simulink model "sbc_uja1169_rw_reg_s32k11x"  (Simulink 9.0)
settings: Solver=FixedStepDiscrete  StartTime=0.0  StopTime=10.0  FixedStep=0.1  RelTol=1e-3  EnableMultiTasking=on
InitFcn:
  | mbd_s32k_consistency_checks(bdroot(gcs));
undefined symbols (not defined in the file): bit, F, LQFP, thumb, UJA1169TK
libraries: mbd_s32k1xx_ec_toolbox x6, mbd_sbc_ec_toolbox x5, simulink x3
Description:
  | This model shows how to use SBC_Read_Register and SBC_Write_Register blocks.
  | The SBC is configured with reset threshold set to 90 % of V1 nominal output voltage, and after several seconds the reset threshold is set to 60% of V1 .
  | 
  | 
  | Validation:
  |  - RED Led should be on about 5 sec (reset threshold set to 90 %)
  | -  BLUE Led should be on after more than 5 sec (reset threshold set to 60 %)
  | 
  | Notes:
  | The test requires correct factory settings: FNMC bit disabled, SBC_UJA_SBC_SDMC_DIS disabled and slpc must be allowed.
  | For running other applications is recommended to move the SBC in FNMC after running this example,
  | otherwise CAN transceiver can be disabled because SBC goes in LIMP mode due to lack of watchdog feed.
  | 
  | To move SBC in FNMC state:
  |    - pin RSTN (TP24) is held LOW
  |    -CANH is pulled up to Vbat
  |    -CANL is pulled down to GND
  | 
  | 
  | HW prerequisite:
  | - S32K116/S32K118
  | - One Power Adapter 12V
settings Model: Creator=NXP MBDT Team  LastModifiedBy=nxf35172
settings DataIOCC: ExternalInput=off  InitialState=off  SaveFormat=Dataset  SaveOutput=off  SignalLogging=off  SaveTime=off
settings OptimizationCC: DefaultParameterBehavior=Inlined  LifeSpan=1
settings DebuggingCC: UnderspecifiedInitializationDetection=Simplified  MergeDetectMultiDrivingBlocksExec=error  InheritedTsInSrcMsg=none  SingleTaskRateTransMsg=error  UnconnectedInputMsg=error  UnconnectedOutputMsg=error  UnconnectedLineMsg=error  UnknownTsInhSupMsg=error
settings HardwareCC: ProdLargestAtomicInteger=Long  ProdLargestAtomicFloat=Double  ProdIntDivRoundTo=Zero  ProdEndianess=LittleEndian  ProdHWDeviceType=ARM Compatible->ARM Cortex
settings ModelReferenceCC: PropagateSignalLabelsOutOfModel=on
settings SFSimCC: MATLABDynamicMemAlloc=off
settings RTWCC: SystemTargetFile=mbd_s32k.tlc  MakeCommand=mbd_s32k_make_rtw COPY_MDLREF_INCLUDES=0  TemplateMakefile=mbd_s32k.tmf  Description=Model Based Design Toolbox S32K14x Code Generation Target  GenerateReport=on  IncludeHyperlinkInReport=on  LaunchReport=on  GenerateTraceInfo=on  GenerateTraceReport=on  GenerateTraceReportSl=on  GenerateTraceReportSf=on  GenerateTraceReportEml=on
settings CodeAppCC: ForceParamTrailComments=on  IgnoreCustomStorageClasses=off  OperatorAnnotations=on  SimulinkDataObjDesc=on  SFDataObjDesc=on  MATLABFcnDesc=on  InsertBlockDesc=on  MATLABSourceComments=on
settings STFCustomTargetCC: CombineOutputUpdateFcns=on  ERTCustomFileBanners=on  SupportContinuousTime=off  SupportNonInlinedSFcns=off  RemoveResetFunc=on  MATLABClassNameForMDSCustomization=Simulink.SoftwareTarget.ERTCustomization  GRTInterface=off  SystemTargetFile=mbd_s32k.tlc
settings ERTTargetCC: MultiwordLength=2048  ParMdlRefBuildCompliant=off  CompOptLevelCompliant=off  ConcurrentExecutionCompliant=off  ModelStepFunctionPrototypeControlCompliant=off  CPPClassGenCompliant=off  UseToolchainInfoCompliant=off  InlinedParameterPlacement=NonHierarchical  ERTCustomFileTemplate=example_file_process.tlc

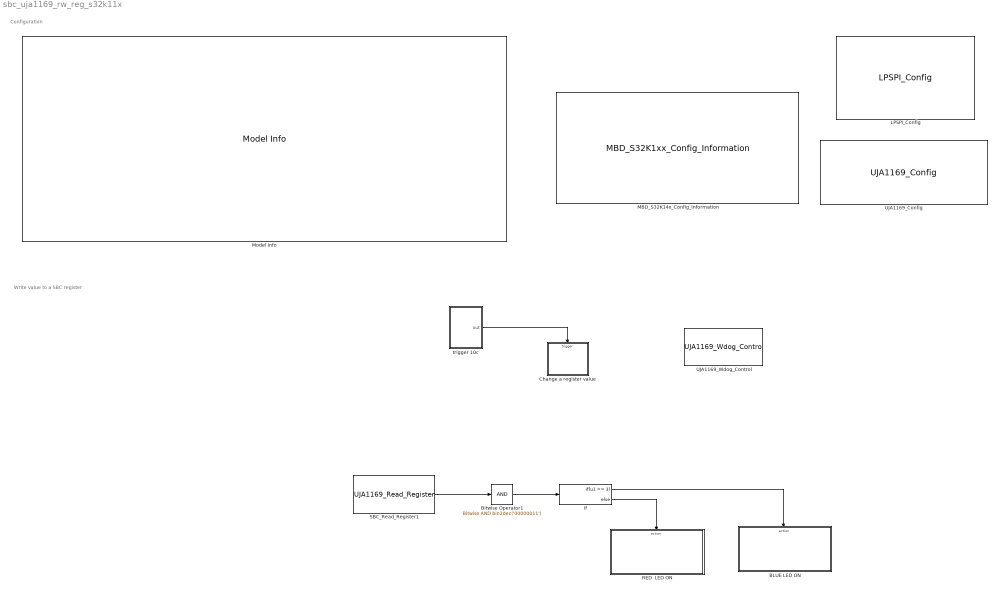
== system sbc_uja1169_rw_reg_s32k11x ==
  note: Configuration
  note: Write value to a SBC register
  BLUE LED ON : Subsystem  TreatAsAtomicUnit=on
  Bitwise Operator1 : simulink/Logic and Bit Operations/Bitwise Operator  logicop=AND  UseBitMask=on  BitMask=bin2dec('00000011')  BitMaskRealWorld=Stored Integer
  Change a register value : Subsystem
  If : If  IfExpression=u1 == 3
  "LPSPI_Config " : mbd_s32k1xx_ec_toolbox/Communication Blocks/SPI Blocks/LPSPI_Config   Priority=1  InstanceNumber=0  Role=Master  BaudRate=50000  ShowAdvanced=on  sin=PTB3: [LPSPI0_SIN | LPSPI Serial Data Input]  sout=PTB4: [LPSPI0_SOUT | LPSPI Serial Data Output]  sck=PTB2: [LPSPI0_SCK | LPSPI Serial Clock I/O]  pcs0=None  pcs1=PTB5: [LPSPI0_PCS1 | Peripheral Chip Select 1]  pcs2=None  pcs3=not available  CPHA=1  CPOL=0  BitOrder=MSB first  TransferSize=16  WhichPCS=1  PCSPol=ActiveLow  ContinuousTransfer=off
  MBD_S32K14x_Config_Information : mbd_s32k1xx_ec_toolbox/MBD_S32K1xx_Config_Information  Priority=0  mbdt_ver=0  disp_str=|  config_params=[]  mcu_target_name=S32K118  mcu_target_package=48-LQFP  mcu_target_sram_size=25KB  mcu_system_clock_freq=40  mcu_xtal_freq=External 40  mcu_steptick_timer=LPIT Channel 0  mcu_steptick_prio=3  ds_import_enable=on  target_compiler=GCC  target_memory=FLASH  gcc_target_compile_opts=-mcpu=cortex-m0plus -mthumb -O1 -g -gstrict-dwarf  gcc_target_assemble_opts=-mcpu=cortex-m0plus -mthumb -g  gcc_target_link_opts=-mcpu=cortex-m0plus -mthumb  gcc_target_default_lcf=on  gcc_target_user_lcf=S32K118_25_flash.ld  ghs_target_compile_opts=-mcpu=cortexm0plus -mthumb -fsoft -Ogeneral -Wundef -Wimplicit-int -Wshadow -Wtrigraphs --no_commons --gnu_asm -gnu99 -gdwarf-2 -G  ghs_target_assemble_opts=-mcpu=cortexm0plus -mthumb -fsoft --gnu_asm  ghs_target_link_opts=-mcpu=cortexm0plus -mthumb -fsoft  ghs_target_default_lcf=off  ghs_target_user_lcf=S32K118_25_flash.ld  iar_target_compile_opts=--thumb -Ol -e --debug --dlib_config normal  iar_target_assemble_opts=--thumb  iar_target_link_opts=--no_exceptions --vfe --inline  iar_target_default_lcf=off  iar_target_user_lcf=S32K118_25_flash.icf  pil_download_enable=off  rbl_download_enable=on  rbl_start_delay=5000000  rbl_download_interface=OpenSDA  rbl_restart_request=off  rbl_com_port=Custom  rbl_com_port_custom=COM1  pil_download_rate=57600  pil_opensda_drive=Custom  pil_opensda_drive_custom=D  pil_uart_instance=0  pil_uart_rx=PTA2: [LPUART0_RX | Receive]  pil_uart_tx=PTA3: [LPUART0_TX | Transmit]  FTM_PWM_PcrCheckEnDis=on  FTM_Input_Edge_Inputs_PcrCheckEnDis=off  FTM_Dual_Edge_Inputs_PcrCheckEnDis=off  FTM_Quadrature_Inputs_PcrCheckEnDis=off  FTM_Hall_Sensor_Inputs_PcrCheckEnDis=on  LPTMR_PcrCheckEnDis=off  PIT_PcrCheckEnDis=off  RTC_PcrCheckEnDis=off  FlexCAN_PcrCheckEnDis=off  LIN_PcrCheckEnDis=on  FlexIO_PcrCheckEnDis=off  LPI2C_PcrCheckEnDis=off  LPSPI_PcrCheckEnDis=on  LPUART_PcrCheckEnDis=off  CMP_PcrCheckEnDis=off  GPIO_OutputPcrCheckEnDis=on  GPIO_InputPcrCheckEnDis=on  SBC_PcrCheckEnDis=on  AMMCLIB_PcrCheckEnDis=off  FM_PcrCheckEnDis=off  Profile_PcrCheckEnDis=off  ConfigParams_PcrCheckEnDis=on  ModelRef_PcrCheckEnDis=on  PDB0_PcrCheckEnDis=off  CSEc_PcrCheckEnDis=off  eDMA_PcrCheckEnDis=off  ADC_PcrCheckEnDis=off  WDOG_PcrCheckEnDis=on
      | Target : S32K144-64KB_SRAM
      | Package : 100-pin
      | System clock : 80 MHz
      | XTAL clock : External 8 MHz
      | Compiler : IAR
      | Target Type : FLASH
      | Download Code after build : off
      | Step Tick Interrupt Priority : 15
  Model Info : simulink/Model-Wide Utilities/Model Info  Frame=off  DisplayStringWithTags=|  HorizontalTextAlignment=Left  LeftAlignmentValue=0.02
      | Model Name: %<ModelName>
      | 
      | Description: %<Description>
  RED  LED ON : Subsystem  TreatAsAtomicUnit=on
  SBC_Read_Register1 : mbd_sbc_ec_toolbox/UJA116x/UJA1169_Read_Register  Priority=4  Register=SBC_UJA_REGULATOR
  UJA1169_Config : mbd_sbc_ec_toolbox/UJA116x/UJA1169_Config  Priority=2  modeCtrl=NORMAL  deviceModel=UJA1169TK/F  LHCtrl=Floating  pdc=higher value  VextConfig=V2C OFF  ResetTresh=90  WdogModeCtrl=Autonomous  NominalPer=128 ms  Lock0=off  Lock1=off  Lock2=off  Lock3=off  Lock4=off  Lock5=off  Lock6=off  FDcontrol=off  FDPartialOK=off  FDPartial=off  CANmodeCtrl=Offline  dataRate=50 kbit/s  ID1=0  ID2=0  ID3=0  ID4=0  IDmask1=0  IDmask2=0  IDmask3=0  IDmask4=0  IdFormat=11-bit  PartialNetwData=Don't care  DataLength=0  dataMask0=0  dataMask4=0  dataMask1=0  dataMask5=0  dataMask2=0  dataMask6=0  dataMask3=0  dataMask7=0  V2overv=on  V2underv=on  V1underv=on  CANsilence=on  CANfailure=on  CANwkUp=on  overtempWrng=on  spiFailure=on  risingEdge=on  fallingEdge=on
  UJA1169_Wdog_Control : mbd_sbc_ec_toolbox/UJA116x/UJA1169_Wdog_Control  reset=on  mode=off  ModeCtrl=Window  period=off  NominalPer=128 ms
  trigger 10c : Stateflow chart  Priority=0  TreatAsAtomicUnit=on
  wires:
  If/1 -> BLUE LED ON/Action
  trigger 10c/1(out) -> Change a register value/Trigger
  Bitwise Operator1/1 -> If/1
  SBC_Read_Register1/1 -> Bitwise Operator1/1
  If/2 -> RED  LED ON/Action

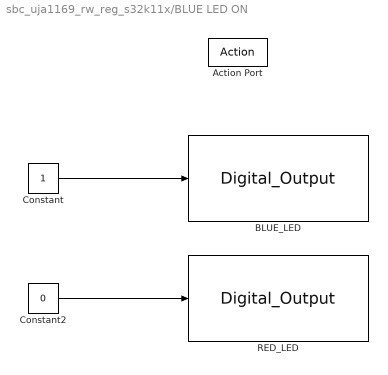
== system sbc_uja1169_rw_reg_s32k11x/BLUE LED ON ==
  Action Port : ActionPort
  BLUE_LED : mbd_s32k1xx_ec_toolbox/GPIO Blocks/Digital_Output  gpio_pin=PTE8: [PTE8 | Port E I/O]  init_val=Low  drive_strength=Low
  Constant : Constant  OutDataTypeStr=boolean
  Constant2 : Constant  Value=0  OutDataTypeStr=boolean
  RED_LED : mbd_s32k1xx_ec_toolbox/GPIO Blocks/Digital_Output  gpio_pin=PTD16: [PTD16 | Port D I/O]  init_val=Low  drive_strength=Low
  wires:
  Constant2/1 -> RED_LED/1
  Constant/1 -> BLUE_LED/1

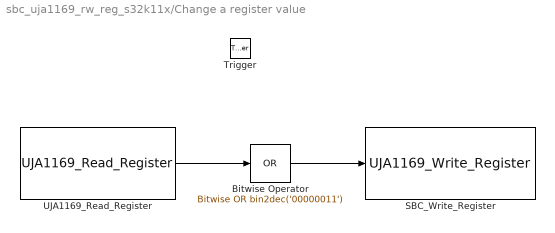
== system sbc_uja1169_rw_reg_s32k11x/Change a register value ==
  Trigger : TriggerPort  VariantControl=Variant
  Bitwise Operator : simulink/Logic and Bit Operations/Bitwise Operator  logicop=OR  UseBitMask=on  BitMask=bin2dec('00000011')  BitMaskRealWorld=Stored Integer
  SBC_Write_Register : mbd_sbc_ec_toolbox/UJA116x/UJA1169_Write_Register  Register=SBC_UJA_REGULATOR
  UJA1169_Read_Register : mbd_sbc_ec_toolbox/UJA116x/UJA1169_Read_Register  Register=SBC_UJA_REGULATOR
  wires:
  UJA1169_Read_Register/1 -> Bitwise Operator/1
  Bitwise Operator/1 -> SBC_Write_Register/1

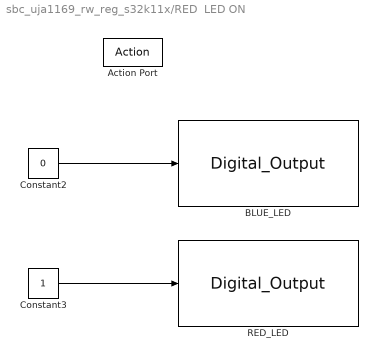
== system sbc_uja1169_rw_reg_s32k11x/RED  LED ON ==
  Action Port : ActionPort
  BLUE_LED : mbd_s32k1xx_ec_toolbox/GPIO Blocks/Digital_Output  gpio_pin=PTE8: [PTE8 | Port E I/O]  init_val=Low  drive_strength=Low
  Constant2 : Constant  Value=0  OutDataTypeStr=boolean
  Constant3 : Constant  OutDataTypeStr=boolean
  RED_LED : mbd_s32k1xx_ec_toolbox/GPIO Blocks/Digital_Output  gpio_pin=PTD16: [PTD16 | Port D I/O]  init_val=Low  drive_strength=Low
  wires:
  Constant2/1 -> BLUE_LED/1
  Constant3/1 -> RED_LED/1

== stateflow chart trigger 10c ==
  settings: executeAtInitialization=1
  state A
    du:
    cnt = cnt +1;
    out = 0;
  state A1
    du:
    cnt = 0;
    out = 1;
  (default) -> A : {cnt = 0;}
  A1 -> A : [cnt == 0]
  A -> A1 : [cnt == 50]
  data: cnt local uint32 =0; out output uint32
